simulink model "model2"  (R2023b)
settings: Solver=VariableStepAuto  StartTime=0.0  StopTime=10.0  RelTol=1e-3
undefined symbols (not defined in the file): b1da, d6e66bc8738b, DiscIntNeverNeededParam, magnitude, Newton, Raphson
libraries: simulink x70, slpidlib x25
(part 1 of 4)
settings Model: Creator=OSCAR4  LastModifiedBy=OSCAR4

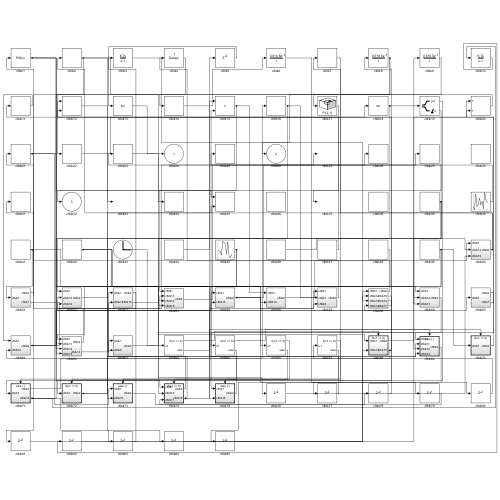
[thumbnail: Simulink's stored preview of the top-level diagram]
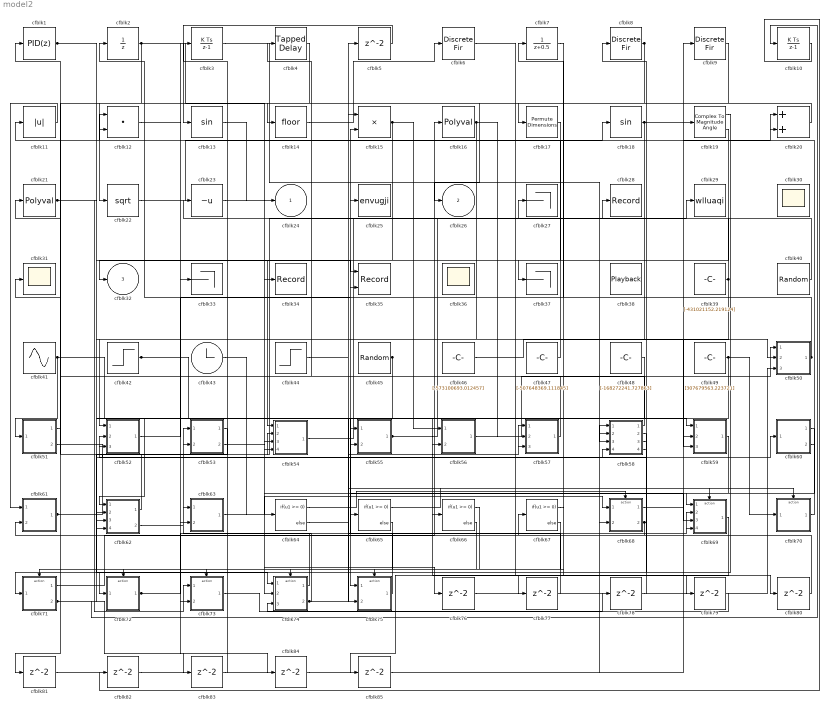
== system model2 ==
  cfblk1 : slpidlib/PID Controller  Controller=PID  Form=Parallel  TimeDomain=Discrete-time  UseExternalTs=off  SampleTime=1  IntegratorMethod=Forward Euler  FilterMethod=Forward Euler  ControllerParametersSource=internal  P=1  I=1  UseKiTs=off  D=0  N=100  UseFilter=on  TunerSelectOption=Transfer Function Based (PID Tuner App)  InitialConditionSource=internal  InitialConditionForIntegrator=0  InitialConditionForFilter=0  DifferentiatorICPrevScaledInput=0  ExternalReset=none  TrackingMode=off  Kt=1  LimitOutput=off  SatLimitsSource=internal  UpperSaturationLimit=inf  LowerSaturationLimit=-inf  LinearizeAsGain=off  AntiWindupMode=none  Kb=1  LimitIntegrator=off  UpperIntegratorSaturationLimit=inf  LowerIntegratorSaturationLimit=-inf  POutMin=[]  POutMax=[]  IOutMin=[]  IOutMax=[]  DOutMin=[]  DOutMax=[]  NOutMin=[]  NOutMax=[]  SumOutMin=[]  SumOutMax=[]  SaturationOutMin=[]  SaturationOutMax=[]  PParamMin=[]  PParamMax=[]  IParamMin=[]  IParamMax=[]  DParamMin=[]  DParamMax=[]  NParamMin=[]  NParamMax=[]  KbParamMin=[]  KbParamMax=[]  KtParamMin=[]  KtParamMax=[]  KbOutMin=[]  KbOutMax=[]  KtOutMin=[]  KtOutMax=[]  IntegratorOutMin=[]  IntegratorOutMax=[]  FilterOutMin=[]  FilterOutMax=[]  SumI1OutMin=[]  SumI1OutMax=[]  SumI2OutMin=[]  SumI2OutMax=[]  SumI3OutMin=[]  SumI3OutMax=[]  SumI4OutMin=[]  SumI4OutMax=[]  SumDOutMin=[]  SumDOutMax=[]  DifferentiatorOutMin=[]  DifferentiatorOutMax=[]  FilterDiffOutCoefMin=[]  FilterDiffOutCoefMax=[]  ReciprocalOutMin=[]  ReciprocalOutMax=[]  SumDenOutMin=[]  SumDenOutMax=[]  SumNumOutMin=[]  SumNumOutMax=[]  DivideOutMin=[]  DivideOutMax=[]  UdiffTsProdOutMin=[]  UdiffTsProdOutMax=[]  NTsProdOutMin=[]  NTsProdOutMax=[]  UintegralTsProdOutMin=[]  UintegralTsProdOutMax=[]  UngainTsProdOutMin=[]  UngainTsProdOutMax=[]  ClampingZeroOutDataTypeStr=Inherit: Inherit via back propagation  ClampingZeroOutMin=[]  ClampingZeroOutMax=[]  FilterDenConstantOutDataTypeStr=Inherit: Inherit via back propagation  FilterDenConstantOutMin=[]  FilterDenConstantOutMax=[]  PCopyOutDataTypeStr=Inherit: Inherit via back propagation  PCopyOutMin=[]  PCopyOutMax=[]  NCopyOutDataTypeStr=Inherit: Inherit via back propagation  NCopyOutMin=[]  NCopyOutMax=[]  IntegratorContinuousStateAttributes=''  IntegratorStateMustResolveToSignalObject=off  IntegratorRTWStateStorageClass=Auto  FilterContinuousStateAttributes=''  FilterStateMustResolveToSignalObject=off  FilterRTWStateStorageClass=Auto  ParallelPVariant=InternalParameters  IdealPVariant=Disabled  IVariant=InternalParameters  DVariant=InternalParameters  IntegratorVariant=Discrete  SatVariant=Disabled  AWVariant=Passthrough  PCopyVariant=Disabled  TRVariant=Disabled  FdbkBlocksVariant=Forward  IdealPFdbkVariant=Disabled  SatFdbkVariant=Disabled  DerivativeFilterVariant=ForwardEulerFilter  NVariant=InternalParameters  NCopyVariant=Disabled  FilterICVariant=InternalICsFilter  IntegratorICVariant=InternalICs  ExternalResetVariant=Disabled  TRSumVariant=Passthrough  SumFdbkVariant=Disabled  SumVariant=Sum_PID  TsampFilterVariant=InternalTs  TsampNgainVariant=Passthrough  TsampIntegralVariant=Disabled_SignalSpec  ExternalSaturationOutDataTypeStr=Inherit: Same as second input
      settings: LibrarySourceBlock=simulink/Discrete/Discrete PID Controller
  cfblk10 : DiscreteIntegrator  ICPrevOutput=DiscIntNeverNeededParam  ICPrevScaledInput=DiscIntNeverNeededParam
  cfblk11 : Abs  SaturateOnIntegerOverflow=off
  cfblk12 : DotProduct  OutDataTypeStr=Inherit: Inherit via internal rule
  cfblk13 : Trigonometry
  cfblk14 : Rounding
  cfblk15 : Product
  cfblk16 : Polyval  Coefs=[ +2.081618890e-019, -1.441693666e-014, +4.719686976e-010, -8.536869453e-006, +1.621573104e-001, -8.087801117e+001 ]
  cfblk17 : PermuteDimensions
  cfblk18 : Trigonometry
  cfblk19 : ComplexToMagnitudeAngle
  cfblk2 : UnitDelay  HasFrameUpgradeWarning=on
  cfblk20 : Sum
  cfblk21 : Polyval  Coefs=[ +2.081618890e-019, -1.441693666e-014, +4.719686976e-010, -8.536869453e-006, +1.621573104e-001, -8.087801117e+001 ]
  cfblk22 : Sqrt
  cfblk23 : UnaryMinus
  cfblk25 : ToWorkspace  VariableName=envugji  SaveFormat=Timeseries  SampleTime=-1
  cfblk27 : Terminator
  cfblk28 : Record  FileSettingsInternal="{\"entries\":[{\"content\":{\"excelSettings\":{\"content\":{},\"type\":\"Streamout.ExcelSettings\"}},\"type\":\"Streamout.FileSettingStorage\",\"uuid\":\"\"}],\"packageUris\":[\"http:\\/\\/schema.mathworks.com\\/mf0\\/streamout_blocks\\/R2020a\"],\"version\":\"1.0\"}"  SignalsInternal="{\"entries\":[{\"content\":{\"signals\":[{\"content\":{\"blockPath\":[],\"dimensions\":[1],\"domain\":\"\",\"lineColor\":\"#ff13a6\",\"plots\":[1],\"port\":1,\"sid\":[\"\"],\"signalID\":1141,\"signalName\":\"cfblk55\"},\"type\":\"RecordBlkView.Signal\",\"uuid\":\"\"}]},\"type\":\"RecordBlkView.InputSignals\",\"uuid\":\"\"}],\"packageUris\":[\"http:\\/\\/schema.mathworks.com\\/mf0\\/streamout_blocks\\/R2020a\"],\"version\":\"1.0\"}"  VisualizationBindings="{\"sparklinesplugin\":{\"info\":[{\"bindingParametersList\":[],\"subplotID\":1}]}}"
  cfblk29 : ToWorkspace  VariableName=wlluaqi  SaveFormat=Timeseries  SampleTime=-1
  cfblk3 : DiscreteIntegrator  ICPrevOutput=DiscIntNeverNeededParam  ICPrevScaledInput=DiscIntNeverNeededParam
  cfblk30 : Scope
      settings: Floating=on
  cfblk31 : Scope
  cfblk33 : Terminator
  cfblk34 : Record  FileSettingsInternal="{\"entries\":[{\"content\":{\"excelSettings\":{\"content\":{},\"type\":\"Streamout.ExcelSettings\"}},\"type\":\"Streamout.FileSettingStorage\",\"uuid\":\"\"}],\"packageUris\":[\"http:\\/\\/schema.mathworks.com\\/mf0\\/streamout_blocks\\/R2020a\"],\"version\":\"1.0\"}"  SignalsInternal="{\"entries\":[{\"content\":{\"signals\":[{\"content\":{\"blockPath\":[],\"dimensions\":[1],\"domain\":\"\",\"lineColor\":\"#22b573\",\"plots\":[1],\"port\":1,\"sid\":[\"\"],\"signalID\":1149,\"signalName\":\"cfblk2\"},\"type\":\"RecordBlkView.Signal\",\"uuid\":\"\"}]},\"type\":\"RecordBlkView.InputSignals\",\"uuid\":\"\"}],\"packageUris\":[\"http:\\/\\/schema.mathworks.com\\/mf0\\/streamout_blocks\\/R2020a\"],\"version\":\"1.0\"}"  VisualizationBindings="{\"sparklinesplugin\":{\"info\":[{\"bindingParametersList\":[],\"subplotID\":1}]}}"
  cfblk35 : Record  FileSettingsInternal="{\"entries\":[{\"content\":{\"excelSettings\":{\"content\":{},\"type\":\"Streamout.ExcelSettings\"}},\"type\":\"Streamout.FileSettingStorage\",\"uuid\":\"\"}],\"packageUris\":[\"http:\\/\\/schema.mathworks.com\\/mf0\\/streamout_blocks\\/R2020a\"],\"version\":\"1.0\"}"  Layout=[1 1]  SignalsInternal="{\"entries\":[{\"content\":{\"signals\":[{\"content\":{\"blockPath\":[],\"dimensions\":[1],\"domain\":\"\",\"lineColor\":\"#a2142f\",\"plots\":[1],\"port\":1,\"sid\":[\"\"],\"signalID\":1153,\"signalName\":\"cfblk1\"},\"type\":\"RecordBlkView.Signal\",\"uuid\":\"\"},{\"content\":{\"blockPath\":[],\"dimensions\":[1],\"domain\":\"\",\"lineColor\":\"#139fff\",\"plots\":[1],\"port\":2,\"sid\":[\"\"],\"signalID\":1157,\"signalName\":\"cfblk52\"},\"type\":\"RecordBlkView.Signal\",\"uuid\":\"\"}]},\"type\":\"RecordBlkView.InputSignals\",\"uuid\":\"\"}],\"packageUris\":[\"http:\\/\\/schema.mathworks.com\\/mf0\\/streamout_blocks\\/R2020a\"],\"version\":\"1.0\"}"  VisualizationBindings="{\"xyplotplugin\":{\"info\":[{\"series\":[{\"bindingParametersList\":[{\"parameter\":\"X-Axis\",\"signalID\":1153,\"signalName\":\"cfblk1\"},{\"parameter\":\"Y-Axis\",\"signalID\":1157,\"signalName\":\"cfblk52\"}],\"seriesID\":35529}],\"subplotID\":1}]}}"  CompatibilityTag=XY
  cfblk36 : Scope
      settings: Floating=on
  cfblk37 : Terminator
  cfblk38 : Playback  NumPorts=0  PartName=63b8ea15-6b82-47df-b1da-d6e66bc8738b
  cfblk39 : Constant  Value=[-431021152.219124]  SampleTime=1
  cfblk4 : simulink/Discrete/Tapped Delay  vinit=0.0  samptime=-1  NumDelays=1  DelayOrder=Oldest  includeCurrent=off
  cfblk40 : UniformRandomNumber  Minimum=[-8305883063.476324]  Maximum=[6336167478.410847]  Seed=[29457914.000000]  SampleTime=0.1
  cfblk41 : Sin  Amplitude=[815797185.839253]  Bias=[956764081.088228]  SampleTime=0
  cfblk42 : Step  Time=[20.000000]  Before=[-203811535.519444]  After=[543324155.345459]  SampleTime=0
  cfblk43 : Clock
  cfblk44 : Step  Time=[32.000000]  Before=[-285476932.662708]  After=[117735768.071794]  SampleTime=0
  cfblk45 : RandomNumber  Mean=[37780.519300]  Variance=[5936.131945]  Seed=[246649944.000000]  SampleTime=0.1
  cfblk46 : Constant  Value=[-573100693.012457]  SampleTime=1
  cfblk47 : Constant  Value=[-507648369.111845]  SampleTime=1
  cfblk48 : Constant  Value=[-168272241.727863]  SampleTime=1
  cfblk49 : Constant  Value=[307679563.223721]  SampleTime=1
  cfblk{5,76..85} (11 alike) : Delay  SampleTime=1
  cfblk50 : Subsystem
  cfblk51 : Subsystem
  cfblk52 : Subsystem
  cfblk53 : Subsystem
  cfblk54 : Subsystem
  cfblk55 : Subsystem
  cfblk56 : Subsystem
  cfblk57 : Subsystem
  cfblk58 : Subsystem
  cfblk59 : Subsystem
  cfblk6 : DiscreteFir  SampleTime=1
  cfblk60 : Subsystem
  cfblk61 : Subsystem
  cfblk62 : Subsystem
  cfblk63 : Subsystem
  cfblk{64..67} (4 alike) : If  IfExpression=u1 >= 0  SampleTime=1
  cfblk68 : Subsystem  TreatAsAtomicUnit=on
  cfblk69 : Subsystem  TreatAsAtomicUnit=on
  cfblk7 : DiscreteTransferFcn  SampleTime=1
  cfblk70 : Subsystem  TreatAsAtomicUnit=on
  cfblk71 : Subsystem  TreatAsAtomicUnit=on
  cfblk72 : Subsystem  TreatAsAtomicUnit=on
  cfblk73 : Subsystem  TreatAsAtomicUnit=on
  cfblk74 : Subsystem  TreatAsAtomicUnit=on
  cfblk75 : Subsystem  TreatAsAtomicUnit=on
  cfblk8 : DiscreteFir  SampleTime=1
  cfblk9 : DiscreteFir  SampleTime=1
  cfblk24 : Outport
  cfblk26 : Outport  Port=2
  cfblk32 : Outport  Port=3
  wires:
  cfblk54/1(cfblk2) -> cfblk29/1
  cfblk14/1 -> cfblk6/1
  cfblk19/1 -> cfblk72/1(cfblk1)
  cfblk41/1 -> cfblk51/1(cfblk1), cfblk56/2(cfblk10)
  cfblk13/1 -> cfblk24/1
  cfblk47/1 -> cfblk11/1
  cfblk21/1 -> cfblk73/1(cfblk1), cfblk74/1(cfblk1)
  cfblk71/1(cfblk2) -> cfblk16/1
  cfblk74/1(cfblk2) -> cfblk53/1(cfblk1)
  cfblk43/1 -> cfblk64/1
  cfblk20/1 -> cfblk17/1
  cfblk62/1(cfblk2) -> cfblk31/1
  cfblk59/1(cfblk2) -> cfblk75/1(cfblk1)
  cfblk56/1(cfblk2) -> cfblk50/1(cfblk1)
  cfblk62/2(cfblk14) -> cfblk53/2(cfblk12)
  cfblk5/1 -> cfblk13/1
  cfblk51/1(cfblk2) -> cfblk1/1
  cfblk4/1 -> cfblk22/1
  cfblk17/1 -> cfblk37/1
  cfblk8/1 -> cfblk26/1, cfblk81/1
  cfblk60/1(cfblk2) -> cfblk69/1(cfblk1)
  cfblk75/1(cfblk2) -> cfblk15/2
  cfblk74/2(cfblk12) -> cfblk63/1(cfblk1), cfblk57/1(cfblk1)
  cfblk3/1 -> cfblk58/3(cfblk13)
  cfblk51/2(cfblk7) -> cfblk60/1(cfblk1)
  cfblk18/1 -> cfblk9/1, cfblk62/3(cfblk12)
  cfblk49/1 -> cfblk65/1, cfblk70/1(cfblk1), cfblk54/3(cfblk14)
  cfblk39/1 -> cfblk52/1(cfblk1), cfblk23/1, cfblk54/4(cfblk15), cfblk59/2(cfblk12)
  cfblk40/1 -> cfblk25/1
  cfblk58/1(cfblk2) -> cfblk21/1
  cfblk72/1(cfblk2) -> cfblk69/2(cfblk11), cfblk69/4(cfblk13)
  cfblk60/2(cfblk7) -> cfblk12/1
  cfblk2/1 -> cfblk33/1, cfblk34/1, cfblk62/2(cfblk11)
  cfblk55/1(cfblk2) -> cfblk28/1, cfblk57/3(cfblk8), cfblk79/1
  cfblk50/1(cfblk2) -> cfblk2/1, cfblk7/1
  cfblk44/1 -> cfblk5/1
  cfblk57/1(cfblk2) -> cfblk4/1
  cfblk61/1(cfblk2) -> cfblk27/1, cfblk54/2(cfblk13), cfblk55/2(cfblk13)
  cfblk42/1 -> cfblk75/2(cfblk16), cfblk66/1, cfblk74/2(cfblk10)
  cfblk46/1 -> cfblk50/2(cfblk14)
  cfblk23/1 -> cfblk69/3(cfblk12)
  cfblk58/2(cfblk15) -> cfblk71/1(cfblk1)
  cfblk58/3(cfblk16) -> cfblk52/2(cfblk15)
  cfblk53/1(cfblk2) -> cfblk52/3(cfblk16)
  cfblk68/1(cfblk2) -> cfblk20/1
  cfblk58/4(cfblk17) -> cfblk12/2
  cfblk15/1 -> cfblk32/1, cfblk56/1(cfblk1)
  cfblk48/1 -> cfblk73/2(cfblk10)
  cfblk1/1 -> cfblk35/1, cfblk59/1(cfblk1), cfblk59/3(cfblk13)
  cfblk11/1 -> cfblk61/1(cfblk1)
  cfblk16/1 -> cfblk63/2(cfblk8), cfblk57/2(cfblk7)
  cfblk19/2 -> cfblk54/1(cfblk1)
  cfblk52/1(cfblk2) -> cfblk35/2
  cfblk45/1 -> cfblk62/1(cfblk1), cfblk62/4(cfblk13)
  cfblk9/1 -> cfblk14/1
  cfblk70/1(cfblk2) -> cfblk20/2
  cfblk68/2(cfblk15) -> cfblk61/2(cfblk12), cfblk8/1
  cfblk63/1(cfblk2) -> cfblk68/1(cfblk1)
  cfblk71/2(cfblk14) -> cfblk10/1, cfblk55/1(cfblk1), cfblk83/1
  cfblk22/1 -> cfblk18/1
  cfblk64/1 -> cfblk68/Action
  cfblk64/2 -> cfblk69/Action
  cfblk65/1 -> cfblk70/Action
  cfblk65/2 -> cfblk71/Action
  cfblk66/1 -> cfblk72/Action
  cfblk66/2 -> cfblk73/Action
  cfblk67/1 -> cfblk74/Action
  cfblk67/2 -> cfblk75/Action
  cfblk53/2(cfblk13) -> cfblk76/1
  cfblk76/1 -> cfblk50/3(cfblk15)
  cfblk7/1 -> cfblk77/1
  cfblk77/1 -> cfblk15/1
  cfblk73/1(cfblk2) -> cfblk78/1
  cfblk78/1 -> cfblk58/4(cfblk14)
  cfblk79/1 -> cfblk74/3(cfblk11)
  cfblk6/1 -> cfblk80/1
  cfblk80/1 -> cfblk67/1
  cfblk81/1 -> cfblk68/2(cfblk14)
  cfblk10/1 -> cfblk82/1
  cfblk82/1 -> cfblk58/2(cfblk12)
  cfblk83/1 -> cfblk3/1
  cfblk12/1 -> cfblk84/1
  cfblk84/1 -> cfblk58/1(cfblk1)
  cfblk69/1(cfblk2) -> cfblk85/1
  cfblk85/1 -> cfblk19/1

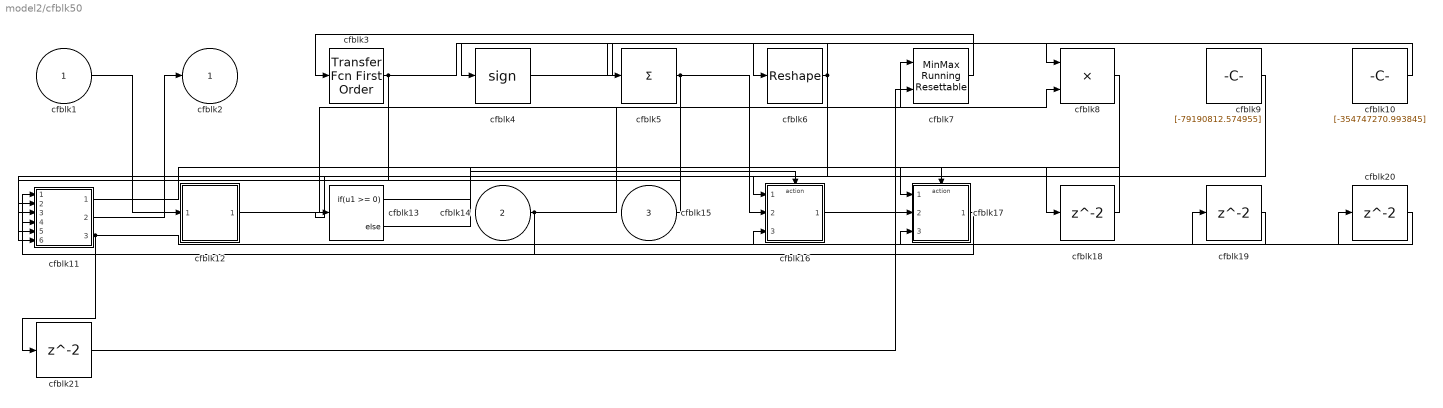
== system model2/cfblk50 ==
  cfblk1 : Inport
  cfblk14 : Inport  Port=2
  cfblk15 : Inport  Port=3
  cfblk10 : Constant  Value=[-354747270.993845]  SampleTime=1
  cfblk11 : Subsystem
  cfblk12 : Subsystem
  cfblk13 : If  IfExpression=u1 >= 0  SampleTime=1
  cfblk16 : Subsystem  TreatAsAtomicUnit=on
  cfblk17 : Subsystem  TreatAsAtomicUnit=on
  cfblk{18..21} (4 alike) : Delay  SampleTime=1
  cfblk3 : simulink/Discrete/Transfer Fcn First Order  PoleZ=0.95  ICPrevOutput=0.0  DoSatur=off
  cfblk4 : Signum
  cfblk5 : Sum  Inputs=+
  cfblk6 : Reshape
  cfblk7 : simulink/Math Operations/MinMax Running Resettable  Function=min  vinit=0.0
  cfblk8 : Product
  cfblk9 : Constant  Value=[-79190812.574955]  SampleTime=1
  cfblk2 : Outport
  wires:
  cfblk1/1 -> cfblk12/1(cfblk1)
  cfblk6/1 -> cfblk4/1, cfblk11/3(cfblk11)
  cfblk12/1(cfblk2) -> cfblk7/1
  cfblk7/1 -> cfblk3/1
  cfblk4/1 -> cfblk8/1
  cfblk10/1 -> cfblk5/1
  cfblk9/1 -> cfblk13/1
  cfblk8/1 -> cfblk16/1(cfblk1)
  cfblk14/1 -> cfblk8/2, cfblk11/4(cfblk12)
  cfblk3/1 -> cfblk6/1, cfblk11/5(cfblk13)
  cfblk17/1(cfblk2) -> cfblk11/1(cfblk1)
  cfblk16/1(cfblk2) -> cfblk17/2(cfblk10)
  cfblk15/1 -> cfblk11/2(cfblk10)
  cfblk5/1 -> cfblk16/2(cfblk10), cfblk11/6(cfblk14)
  cfblk11/2(cfblk15) -> cfblk2/1
  cfblk11/3(cfblk16) -> cfblk19/1, cfblk20/1, cfblk21/1
  cfblk13/1 -> cfblk16/Action
  cfblk13/2 -> cfblk17/Action
  cfblk11/1(cfblk2) -> cfblk18/1
  cfblk18/1 -> cfblk17/1(cfblk1)
  cfblk19/1 -> cfblk16/3(cfblk11)
  cfblk20/1 -> cfblk17/3(cfblk11)
  cfblk21/1 -> cfblk7/2

== system model2/cfblk51 ==
  cfblk1 : Inport
  cfblk3 : Delay  ShowEnablePort=on  SampleTime=1
      settings: InputPortMap=u0,e6
  cfblk4 : Sqrt
  cfblk5 : Sum  Inputs=|++
  cfblk6 : Constant  Value=[536131796.345285]  SampleTime=1
  cfblk8 : Delay  SampleTime=1
  cfblk2 : Outport
  cfblk7 : Outport  Port=2
  wires:
  cfblk6/1 -> cfblk5/1
  cfblk5/1 -> cfblk3/1, cfblk8/1
  cfblk3/1 -> cfblk2/1
  cfblk1/1 -> cfblk3/2
  cfblk4/1 -> cfblk7/1, cfblk5/2
  cfblk8/1 -> cfblk4/1

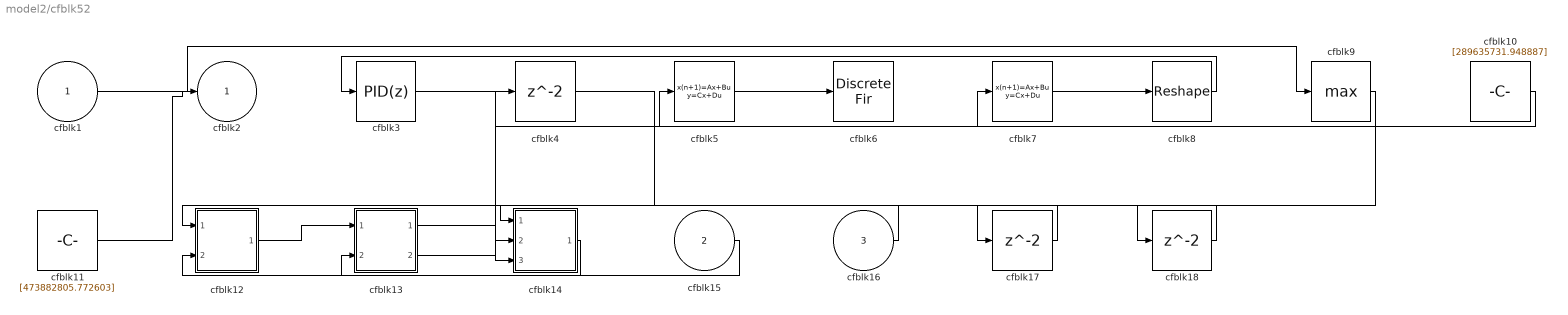
== system model2/cfblk52 ==
  cfblk1 : Inport
  cfblk15 : Inport  Port=2
  cfblk16 : Inport  Port=3
  cfblk10 : Constant  Value=[289635731.948887]  SampleTime=1
  cfblk11 : Constant  Value=[473882805.772603]  SampleTime=1
  cfblk12 : Subsystem
  cfblk13 : Subsystem
  cfblk14 : Subsystem
  cfblk17 : Delay  SampleTime=1
  cfblk18 : Delay  SampleTime=1
  cfblk3 : slpidlib/PID Controller  Controller=PID  Form=Parallel  TimeDomain=Discrete-time  UseExternalTs=off  SampleTime=1  IntegratorMethod=Forward Euler  FilterMethod=Forward Euler  ControllerParametersSource=internal  P=1  I=1  UseKiTs=off  D=0  N=100  UseFilter=on  TunerSelectOption=Transfer Function Based (PID Tuner App)  InitialConditionSource=internal  InitialConditionForIntegrator=0  InitialConditionForFilter=0  DifferentiatorICPrevScaledInput=0  ExternalReset=none  TrackingMode=off  Kt=1  LimitOutput=off  SatLimitsSource=internal  UpperSaturationLimit=inf  LowerSaturationLimit=-inf  LinearizeAsGain=off  AntiWindupMode=none  Kb=1  LimitIntegrator=off  UpperIntegratorSaturationLimit=inf  LowerIntegratorSaturationLimit=-inf  POutMin=[]  POutMax=[]  IOutMin=[]  IOutMax=[]  DOutMin=[]  DOutMax=[]  NOutMin=[]  NOutMax=[]  SumOutMin=[]  SumOutMax=[]  SaturationOutMin=[]  SaturationOutMax=[]  PParamMin=[]  PParamMax=[]  IParamMin=[]  IParamMax=[]  DParamMin=[]  DParamMax=[]  NParamMin=[]  NParamMax=[]  KbParamMin=[]  KbParamMax=[]  KtParamMin=[]  KtParamMax=[]  KbOutMin=[]  KbOutMax=[]  KtOutMin=[]  KtOutMax=[]  IntegratorOutMin=[]  IntegratorOutMax=[]  FilterOutMin=[]  FilterOutMax=[]  SumI1OutMin=[]  SumI1OutMax=[]  SumI2OutMin=[]  SumI2OutMax=[]  SumI3OutMin=[]  SumI3OutMax=[]  SumI4OutMin=[]  SumI4OutMax=[]  SumDOutMin=[]  SumDOutMax=[]  DifferentiatorOutMin=[]  DifferentiatorOutMax=[]  FilterDiffOutCoefMin=[]  FilterDiffOutCoefMax=[]  ReciprocalOutMin=[]  ReciprocalOutMax=[]  SumDenOutMin=[]  SumDenOutMax=[]  SumNumOutMin=[]  SumNumOutMax=[]  DivideOutMin=[]  DivideOutMax=[]  UdiffTsProdOutMin=[]  UdiffTsProdOutMax=[]  NTsProdOutMin=[]  NTsProdOutMax=[]  UintegralTsProdOutMin=[]  UintegralTsProdOutMax=[]  UngainTsProdOutMin=[]  UngainTsProdOutMax=[]  ClampingZeroOutDataTypeStr=Inherit: Inherit via back propagation  ClampingZeroOutMin=[]  ClampingZeroOutMax=[]  FilterDenConstantOutDataTypeStr=Inherit: Inherit via back propagation  FilterDenConstantOutMin=[]  FilterDenConstantOutMax=[]  PCopyOutDataTypeStr=Inherit: Inherit via back propagation  PCopyOutMin=[]  PCopyOutMax=[]  NCopyOutDataTypeStr=Inherit: Inherit via back propagation  NCopyOutMin=[]  NCopyOutMax=[]  IntegratorContinuousStateAttributes=''  IntegratorStateMustResolveToSignalObject=off  IntegratorRTWStateStorageClass=Auto  FilterContinuousStateAttributes=''  FilterStateMustResolveToSignalObject=off  FilterRTWStateStorageClass=Auto  ParallelPVariant=InternalParameters  IdealPVariant=Disabled  IVariant=InternalParameters  DVariant=InternalParameters  IntegratorVariant=Discrete  SatVariant=Disabled  AWVariant=Passthrough  PCopyVariant=Disabled  TRVariant=Disabled  FdbkBlocksVariant=Forward  IdealPFdbkVariant=Disabled  SatFdbkVariant=Disabled  DerivativeFilterVariant=ForwardEulerFilter  NVariant=InternalParameters  NCopyVariant=Disabled  FilterICVariant=InternalICsFilter  IntegratorICVariant=InternalICs  ExternalResetVariant=Disabled  TRSumVariant=Passthrough  SumFdbkVariant=Disabled  SumVariant=Sum_PID  TsampFilterVariant=InternalTs  TsampNgainVariant=Passthrough  TsampIntegralVariant=Disabled_SignalSpec  ExternalSaturationOutDataTypeStr=Inherit: Same as second input
      settings: LibrarySourceBlock=simulink/Discrete/Discrete PID Controller
  cfblk4 : Delay  SampleTime=1
  cfblk5 : DiscreteStateSpace
  cfblk6 : DiscreteFir  SampleTime=1
  cfblk7 : DiscreteStateSpace
  cfblk8 : Reshape
  cfblk9 : MinMax  Function=max
  cfblk2 : Outport
  wires:
  cfblk16/1 -> cfblk12/1(cfblk1)
  cfblk8/1 -> cfblk3/1
  cfblk5/1 -> cfblk6/1
  cfblk7/1 -> cfblk8/1
  cfblk12/1(cfblk2) -> cfblk13/1(cfblk1)
  cfblk1/1 -> cfblk9/1
  cfblk10/1 -> cfblk5/1
  cfblk9/1 -> cfblk14/3(cfblk9)
  cfblk11/1 -> cfblk2/1
  cfblk14/1(cfblk2) -> cfblk12/2(cfblk7)
  cfblk15/1 -> cfblk13/2(cfblk13)
  cfblk13/1(cfblk2) -> cfblk4/1
  cfblk13/2(cfblk14) -> cfblk7/1
  cfblk4/1 -> cfblk17/1
  cfblk17/1 -> cfblk14/2(cfblk8)
  cfblk3/1 -> cfblk18/1
  cfblk18/1 -> cfblk14/1(cfblk1)

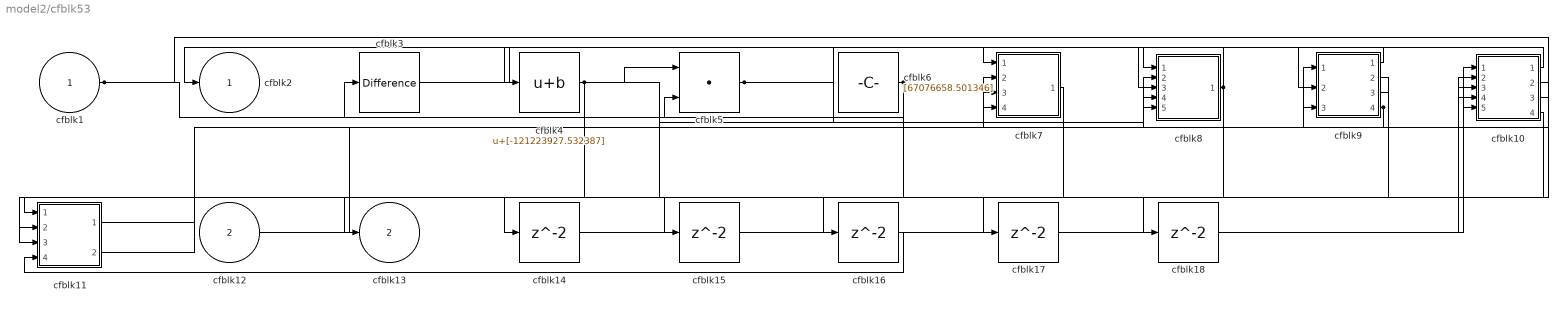
== system model2/cfblk53 ==
  cfblk1 : Inport
  cfblk12 : Inport  Port=2
  cfblk10 : Subsystem
  cfblk11 : Subsystem
  cfblk{14..18} (5 alike) : Delay  SampleTime=1
  cfblk3 : simulink/Discrete/Difference  ICPrevInput=0.0  OutMin=[]  OutMax=[]  OutDataTypeStr=Inherit: Inherit via back propagation  OutDataType=fixdt(1, 16)  OutScaling=2^-10  DoSatur=off
  cfblk4 : Bias  Bias=[-121223927.532387]  SaturateOnIntegerOverflow=off
  cfblk5 : DotProduct  OutDataTypeStr=Inherit: Inherit via internal rule
  cfblk6 : Constant  Value=[67076658.501346]  SampleTime=1
  cfblk7 : Subsystem
  cfblk8 : Subsystem
  cfblk9 : Subsystem
  cfblk2 : Outport
  cfblk13 : Outport  Port=2
  wires:
  cfblk4/1 -> cfblk5/1, cfblk13/1, cfblk8/4(cfblk7), cfblk17/1
  cfblk12/1 -> cfblk9/1(cfblk1)
  cfblk8/1(cfblk2) -> cfblk2/1, cfblk16/1
  cfblk10/1(cfblk2) -> cfblk7/1(cfblk1)
  cfblk6/1 -> cfblk3/1, cfblk11/3(cfblk13)
  cfblk3/1 -> cfblk9/2(cfblk13)
  cfblk1/1 -> cfblk10/1(cfblk1), cfblk5/2
  cfblk10/2(cfblk15) -> cfblk11/1(cfblk1)
  cfblk10/3(cfblk16) -> cfblk7/2(cfblk13)
  cfblk5/1 -> cfblk8/1(cfblk1), cfblk8/3(cfblk6), cfblk8/5(cfblk8)
  cfblk11/2(cfblk15) -> cfblk9/3(cfblk14)
  cfblk10/4(cfblk17) -> cfblk11/2(cfblk12)
  cfblk9/1(cfblk2) -> cfblk4/1
  cfblk9/3(cfblk16) -> cfblk7/3(cfblk14)
  cfblk9/4(cfblk17) -> cfblk8/2(cfblk5), cfblk7/4(cfblk15)
  cfblk7/1(cfblk2) -> cfblk14/1
  cfblk14/1 -> cfblk10/2(cfblk11)
  cfblk11/1(cfblk2) -> cfblk15/1
  cfblk15/1 -> cfblk10/3(cfblk12)
  cfblk16/1 -> cfblk11/4(cfblk14)
  cfblk17/1 -> cfblk10/5(cfblk14)
  cfblk9/2(cfblk15) -> cfblk18/1
  cfblk18/1 -> cfblk10/4(cfblk13)

== system model2/cfblk54 ==
  cfblk1 : Inport
  cfblk13 : Inport  Port=2
  cfblk14 : Inport  Port=3
  cfblk15 : Inport  Port=4
  cfblk10 : Subsystem
  cfblk11 : Subsystem
  cfblk12 : Subsystem
  cfblk16 : Delay  SampleTime=1
  cfblk17 : Delay  SampleTime=1
  cfblk3 : DiscreteStateSpace
  cfblk4 : simulink/Discrete/Transfer Fcn Lead or Lag  PoleZ=0.95  ZeroZ=0.75  ICPrevOutput=0.0  ICPrevInput=0.0  DoSatur=off
  cfblk5 : Trigonometry
  cfblk6 : ComplexToRealImag
  cfblk7 : Constant  Value=[-514549736.041754]  SampleTime=1
  cfblk8 : Subsystem
  cfblk9 : Subsystem
  cfblk2 : Outport
  wires:
  cfblk13/1 -> cfblk3/1
  cfblk10/1(cfblk2) -> cfblk5/1
  cfblk5/1 -> cfblk6/1
  cfblk1/1 -> cfblk12/1(cfblk1)
  cfblk4/1 -> cfblk8/1(cfblk1)
  cfblk12/1(cfblk2) -> cfblk10/2(cfblk8)
  cfblk11/1(cfblk2) -> cfblk9/1(cfblk1)
  cfblk3/1 -> cfblk9/2(cfblk7)
  cfblk6/1 -> cfblk11/1(cfblk1)
  cfblk6/2 -> cfblk2/1
  cfblk11/2(cfblk16) -> cfblk9/3(cfblk8)
  cfblk14/1 -> cfblk12/2(cfblk7)
  cfblk15/1 -> cfblk9/4(cfblk9)
  cfblk7/1 -> cfblk11/2(cfblk14)
  cfblk12/2(cfblk8) -> cfblk11/3(cfblk15)
  cfblk9/1(cfblk2) -> cfblk16/1
  cfblk16/1 -> cfblk10/1(cfblk1)
  cfblk8/1(cfblk2) -> cfblk17/1
  cfblk17/1 -> cfblk4/1

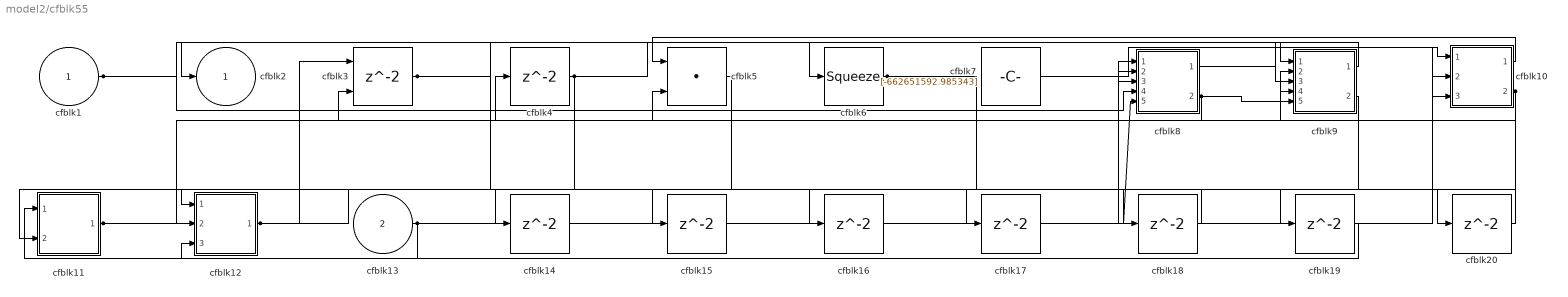
== system model2/cfblk55 ==
  cfblk1 : Inport
  cfblk13 : Inport  Port=2
  cfblk10 : Subsystem
  cfblk11 : Subsystem
  cfblk12 : Subsystem
  cfblk{4,14..20} (8 alike) : Delay  SampleTime=1
  cfblk3 : Delay  ShowEnablePort=on  SampleTime=1
      settings: InputPortMap=u0,e6
  cfblk5 : DotProduct  OutDataTypeStr=Inherit: Inherit via internal rule
  cfblk6 : Squeeze
  cfblk7 : Constant  Value=[-662651592.985343]  SampleTime=1
  cfblk8 : Subsystem
  cfblk9 : Subsystem
  cfblk2 : Outport
  wires:
  cfblk7/1 -> cfblk10/1(cfblk1)
  cfblk6/1 -> cfblk18/1, cfblk19/1
  cfblk10/1(cfblk2) -> cfblk5/1
  cfblk11/1(cfblk2) -> cfblk9/4(cfblk10), cfblk20/1
  cfblk4/1 -> cfblk9/1(cfblk1), cfblk11/2(cfblk8)
  cfblk9/1(cfblk2) -> cfblk2/1
  cfblk8/1(cfblk2) -> cfblk10/3(cfblk12)
  cfblk10/2(cfblk13) -> cfblk9/2(cfblk8), cfblk12/2(cfblk12), cfblk3/2
  cfblk8/2(cfblk16) -> cfblk5/2, cfblk9/5(cfblk11)
  cfblk12/1(cfblk2) -> cfblk3/1, cfblk16/1
  cfblk3/1 -> cfblk6/1, cfblk17/1
  cfblk13/1 -> cfblk11/1(cfblk1), cfblk8/5(cfblk15)
  cfblk1/1 -> cfblk8/4(cfblk14), cfblk9/3(cfblk9)
  cfblk5/1 -> cfblk14/1
  cfblk14/1 -> cfblk10/2(cfblk11)
  cfblk9/2(cfblk12) -> cfblk15/1
  cfblk15/1 -> cfblk8/3(cfblk13)
  cfblk16/1 -> cfblk8/1(cfblk1)
  cfblk17/1 -> cfblk8/2(cfblk12)
  cfblk18/1 -> cfblk12/1(cfblk1)
  cfblk19/1 -> cfblk12/3(cfblk13)
  cfblk20/1 -> cfblk4/1

== system model2/cfblk56 ==
  cfblk1 : Inport
  cfblk10 : Inport  Port=2
  cfblk{11..14} (4 alike) : Delay  SampleTime=1
  cfblk3 : DiscreteFir  SampleTime=1
  cfblk4 : Rounding
  cfblk5 : Sin  TimeSource=Use external signal  SampleTime=0
  cfblk6 : Assignment  DiagnosticForDimensions=Warning  IndexOptions=Index vector (dialog)  Indices=1  OutputSizes=1
  cfblk7 : Polyval  Coefs=[ +2.081618890e-019, -1.441693666e-014, +4.719686976e-010, -8.536869453e-006, +1.621573104e-001, -8.087801117e+001 ]
  cfblk8 : Subsystem
  cfblk9 : Subsystem
  cfblk2 : Outport
  wires:
  cfblk4/1 -> cfblk6/1, cfblk12/1, cfblk13/1
  cfblk10/1 -> cfblk2/1
  cfblk8/1(cfblk2) -> cfblk5/1
  cfblk7/1 -> cfblk3/1, cfblk8/3(cfblk8)
  cfblk1/1 -> cfblk7/1
  cfblk5/1 -> cfblk4/1
  cfblk9/1(cfblk2) -> cfblk6/2
  cfblk3/1 -> cfblk9/2(cfblk6), cfblk8/5(cfblk10)
  cfblk9/2(cfblk8) -> cfblk8/1(cfblk1), cfblk8/6(cfblk11)
  cfblk6/1 -> cfblk11/1
  cfblk11/1 -> cfblk9/1(cfblk1)
  cfblk12/1 -> cfblk8/2(cfblk7)
  cfblk13/1 -> cfblk8/4(cfblk9)
  cfblk8/2(cfblk12) -> cfblk14/1
  cfblk14/1 -> cfblk9/3(cfblk7)

== system model2/cfblk57 ==
  cfblk1 : Inport
  cfblk7 : Inport  Port=2
  cfblk8 : Inport  Port=3
  cfblk10 : Subsystem  TreatAsAtomicUnit=on
  cfblk{11..15} (5 alike) : Delay  SampleTime=1
  cfblk3 : Product  Inputs=*
  cfblk4 : Subsystem
  cfblk5 : Subsystem
  cfblk6 : If  IfExpression=u1 >= 0  SampleTime=1
  cfblk9 : Subsystem  TreatAsAtomicUnit=on
  cfblk2 : Outport
  wires:
  cfblk8/1 -> cfblk2/1, cfblk5/3(cfblk12)
  cfblk1/1 -> cfblk5/1(cfblk1)
  cfblk9/1(cfblk2) -> cfblk10/1(cfblk1)
  cfblk7/1 -> cfblk9/2(cfblk9)
  cfblk10/1(cfblk2) -> cfblk3/1, cfblk11/1, cfblk15/1
  cfblk3/1 -> cfblk4/1(cfblk1), cfblk4/3(cfblk7), cfblk4/6(cfblk10)
  cfblk5/1(cfblk2) -> cfblk9/4(cfblk11)
  cfblk5/2(cfblk14) -> cfblk10/3(cfblk11)
  cfblk5/3(cfblk15) -> cfblk6/1, cfblk4/2(cfblk6), cfblk4/4(cfblk8), cfblk4/5(cfblk9)
  cfblk6/1 -> cfblk9/Action
  cfblk6/2 -> cfblk10/Action
  cfblk11/1 -> cfblk9/3(cfblk10)
  cfblk4/1(cfblk2) -> cfblk12/1
  cfblk12/1 -> cfblk9/1(cfblk1)
  cfblk4/2(cfblk11) -> cfblk13/1
  cfblk13/1 -> cfblk10/2(cfblk10)
  cfblk4/3(cfblk12) -> cfblk14/1
  cfblk14/1 -> cfblk5/2(cfblk11)
  cfblk15/1 -> cfblk5/4(cfblk13)

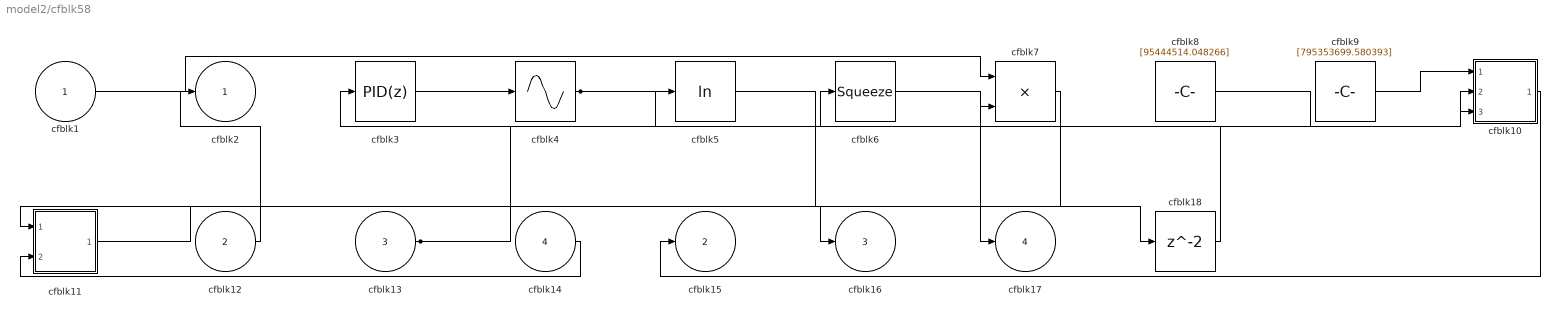
== system model2/cfblk58 ==
  cfblk1 : Inport
  cfblk12 : Inport  Port=2
  cfblk13 : Inport  Port=3
  cfblk14 : Inport  Port=4
  cfblk10 : Subsystem
  cfblk11 : Subsystem
  cfblk18 : Delay  SampleTime=1
  cfblk3 : slpidlib/PID Controller  Controller=PID  Form=Parallel  TimeDomain=Discrete-time  UseExternalTs=off  SampleTime=1  IntegratorMethod=Forward Euler  FilterMethod=Forward Euler  ControllerParametersSource=internal  P=1  I=1  UseKiTs=off  D=0  N=100  UseFilter=on  TunerSelectOption=Transfer Function Based (PID Tuner App)  InitialConditionSource=internal  InitialConditionForIntegrator=0  InitialConditionForFilter=0  DifferentiatorICPrevScaledInput=0  ExternalReset=none  TrackingMode=off  Kt=1  LimitOutput=off  SatLimitsSource=internal  UpperSaturationLimit=inf  LowerSaturationLimit=-inf  LinearizeAsGain=off  AntiWindupMode=none  Kb=1  LimitIntegrator=off  UpperIntegratorSaturationLimit=inf  LowerIntegratorSaturationLimit=-inf  POutMin=[]  POutMax=[]  IOutMin=[]  IOutMax=[]  DOutMin=[]  DOutMax=[]  NOutMin=[]  NOutMax=[]  SumOutMin=[]  SumOutMax=[]  SaturationOutMin=[]  SaturationOutMax=[]  PParamMin=[]  PParamMax=[]  IParamMin=[]  IParamMax=[]  DParamMin=[]  DParamMax=[]  NParamMin=[]  NParamMax=[]  KbParamMin=[]  KbParamMax=[]  KtParamMin=[]  KtParamMax=[]  KbOutMin=[]  KbOutMax=[]  KtOutMin=[]  KtOutMax=[]  IntegratorOutMin=[]  IntegratorOutMax=[]  FilterOutMin=[]  FilterOutMax=[]  SumI1OutMin=[]  SumI1OutMax=[]  SumI2OutMin=[]  SumI2OutMax=[]  SumI3OutMin=[]  SumI3OutMax=[]  SumI4OutMin=[]  SumI4OutMax=[]  SumDOutMin=[]  SumDOutMax=[]  DifferentiatorOutMin=[]  DifferentiatorOutMax=[]  FilterDiffOutCoefMin=[]  FilterDiffOutCoefMax=[]  ReciprocalOutMin=[]  ReciprocalOutMax=[]  SumDenOutMin=[]  SumDenOutMax=[]  SumNumOutMin=[]  SumNumOutMax=[]  DivideOutMin=[]  DivideOutMax=[]  UdiffTsProdOutMin=[]  UdiffTsProdOutMax=[]  NTsProdOutMin=[]  NTsProdOutMax=[]  UintegralTsProdOutMin=[]  UintegralTsProdOutMax=[]  UngainTsProdOutMin=[]  UngainTsProdOutMax=[]  ClampingZeroOutDataTypeStr=Inherit: Inherit via back propagation  ClampingZeroOutMin=[]  ClampingZeroOutMax=[]  FilterDenConstantOutDataTypeStr=Inherit: Inherit via back propagation  FilterDenConstantOutMin=[]  FilterDenConstantOutMax=[]  PCopyOutDataTypeStr=Inherit: Inherit via back propagation  PCopyOutMin=[]  PCopyOutMax=[]  NCopyOutDataTypeStr=Inherit: Inherit via back propagation  NCopyOutMin=[]  NCopyOutMax=[]  IntegratorContinuousStateAttributes=''  IntegratorStateMustResolveToSignalObject=off  IntegratorRTWStateStorageClass=Auto  FilterContinuousStateAttributes=''  FilterStateMustResolveToSignalObject=off  FilterRTWStateStorageClass=Auto  ParallelPVariant=InternalParameters  IdealPVariant=Disabled  IVariant=InternalParameters  DVariant=InternalParameters  IntegratorVariant=Discrete  SatVariant=Disabled  AWVariant=Passthrough  PCopyVariant=Disabled  TRVariant=Disabled  FdbkBlocksVariant=Forward  IdealPFdbkVariant=Disabled  SatFdbkVariant=Disabled  DerivativeFilterVariant=ForwardEulerFilter  NVariant=InternalParameters  NCopyVariant=Disabled  FilterICVariant=InternalICsFilter  IntegratorICVariant=InternalICs  ExternalResetVariant=Disabled  TRSumVariant=Passthrough  SumFdbkVariant=Disabled  SumVariant=Sum_PID  TsampFilterVariant=InternalTs  TsampNgainVariant=Passthrough  TsampIntegralVariant=Disabled_SignalSpec  ExternalSaturationOutDataTypeStr=Inherit: Same as second input
      settings: LibrarySourceBlock=simulink/Discrete/Discrete PID Controller
  cfblk4 : Sin  TimeSource=Use external signal  SampleTime=0
  cfblk5 : Math  Operator=log
  cfblk6 : Squeeze
  cfblk7 : Product
  cfblk8 : Constant  Value=[95444514.048266]  SampleTime=1
  cfblk9 : Constant  Value=[795353699.580393]  SampleTime=1
  cfblk2 : Outport
  cfblk15 : Outport  Port=2
  cfblk16 : Outport  Port=3
  cfblk17 : Outport  Port=4
  wires:
  cfblk7/1 -> cfblk11/1(cfblk1)
  cfblk10/1(cfblk2) -> cfblk15/1
  cfblk14/1 -> cfblk11/2(cfblk8)
  cfblk6/1 -> cfblk17/1
  cfblk3/1 -> cfblk4/1
  cfblk9/1 -> cfblk10/1(cfblk1)
  cfblk1/1 -> cfblk7/1
  cfblk12/1 -> cfblk2/1
  cfblk4/1 -> cfblk5/1, cfblk7/2
  cfblk11/1(cfblk2) -> cfblk16/1
  cfblk8/1 -> cfblk10/2(cfblk14)
  cfblk13/1 -> cfblk10/3(cfblk15), cfblk6/1
  cfblk5/1 -> cfblk18/1
  cfblk18/1 -> cfblk3/1

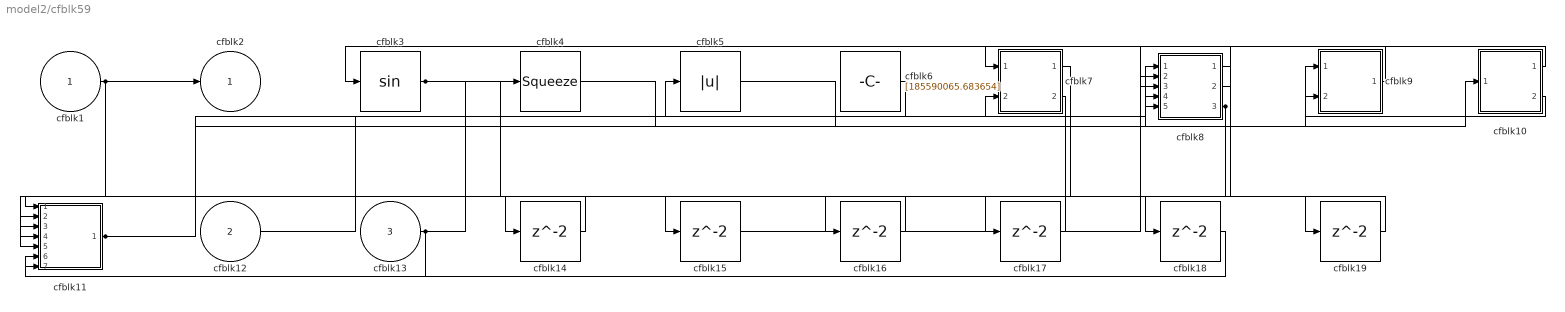
== system model2/cfblk59 ==
  cfblk1 : Inport
  cfblk12 : Inport  Port=2
  cfblk13 : Inport  Port=3
  cfblk10 : Subsystem
  cfblk11 : Subsystem
  cfblk{14..19} (6 alike) : Delay  SampleTime=1
  cfblk3 : Trigonometry
  cfblk4 : Squeeze
  cfblk5 : Abs  SaturateOnIntegerOverflow=off
  cfblk6 : Constant  Value=[185590065.683654]  SampleTime=1
  cfblk7 : Subsystem
  cfblk8 : Subsystem
  cfblk9 : Subsystem
  cfblk2 : Outport
  wires:
  cfblk13/1 -> cfblk4/1, cfblk11/6(cfblk13)
  cfblk1/1 -> cfblk2/1, cfblk11/5(cfblk12)
  cfblk10/1(cfblk2) -> cfblk3/1
  cfblk6/1 -> cfblk5/1
  cfblk10/2(cfblk8) -> cfblk9/1(cfblk1)
  cfblk4/1 -> cfblk8/1(cfblk1)
  cfblk5/1 -> cfblk9/2(cfblk11)
  cfblk9/1(cfblk2) -> cfblk8/3(cfblk12)
  cfblk8/2(cfblk15) -> cfblk7/1(cfblk1)
  cfblk11/1(cfblk2) -> cfblk8/4(cfblk13), cfblk10/1(cfblk1)
  cfblk8/3(cfblk16) -> cfblk17/1, cfblk18/1
  cfblk12/1 -> cfblk8/5(cfblk14)
  cfblk3/1 -> cfblk7/2(cfblk12), cfblk19/1
  cfblk8/1(cfblk2) -> cfblk14/1
  cfblk14/1 -> cfblk11/1(cfblk1)
  cfblk7/1(cfblk2) -> cfblk15/1
  cfblk15/1 -> cfblk8/2(cfblk11)
  cfblk7/2(cfblk13) -> cfblk16/1
  cfblk16/1 -> cfblk11/2(cfblk9)
  cfblk17/1 -> cfblk11/3(cfblk10)
  cfblk18/1 -> cfblk11/7(cfblk14)
  cfblk19/1 -> cfblk11/4(cfblk11)

== system model2/cfblk60 ==
  cfblk1 : Inport
  cfblk3 : UnitDelay  HasFrameUpgradeWarning=on
  cfblk4 : Abs  SaturateOnIntegerOverflow=off
  cfblk5 : simulink/Math Operations/Slider Gain  gain=1  low=0  high=2
  cfblk6 : Subsystem
  cfblk8 : Delay  SampleTime=1
  cfblk2 : Outport
  cfblk7 : Outport  Port=2
  wires:
  cfblk5/1 -> cfblk7/1
  cfblk1/1 -> cfblk5/1, cfblk6/2(cfblk12)
  cfblk6/1(cfblk2) -> cfblk3/1
  cfblk6/2(cfblk13) -> cfblk2/1
  cfblk3/1 -> cfblk4/1
  cfblk4/1 -> cfblk8/1
  cfblk8/1 -> cfblk6/1(cfblk1)

== system model2/cfblk61 ==
  cfblk1 : Inport
  cfblk12 : Inport  Port=2
  cfblk10 : Constant  Value=[389037315.752305]  SampleTime=1
  cfblk11 : Subsystem
  cfblk3 : simulink/Discrete/Difference  ICPrevInput=0.0  OutMin=[]  OutMax=[]  OutDataTypeStr=Inherit: Inherit via back propagation  OutDataType=fixdt(1, 16)  OutScaling=2^-10  DoSatur=off
  cfblk4 : DiscreteIntegrator  ICPrevOutput=DiscIntNeverNeededParam  ICPrevScaledInput=DiscIntNeverNeededParam
  cfblk5 : Abs  SaturateOnIntegerOverflow=off
  cfblk6 : Polyval  Coefs=[ +2.081618890e-019, -1.441693666e-014, +4.719686976e-010, -8.536869453e-006, +1.621573104e-001, -8.087801117e+001 ]
  cfblk7 : Sum  Inputs=+-
  cfblk8 : Abs  SaturateOnIntegerOverflow=off
  cfblk9 : Product  Inputs=**
  cfblk2 : Outport
  wires:
  cfblk1/1 -> cfblk8/1
  cfblk6/1 -> cfblk5/1
  cfblk10/1 -> cfblk6/1
  cfblk12/1 -> cfblk7/1, cfblk7/2
  cfblk4/1 -> cfblk9/1
  cfblk3/1 -> cfblk4/1
  cfblk5/1 -> cfblk3/1
  cfblk8/1 -> cfblk11/1(cfblk1), cfblk11/3(cfblk8)
  cfblk11/1(cfblk2) -> cfblk9/2
  cfblk7/1 -> cfblk11/2(cfblk7), cfblk11/4(cfblk9)
  cfblk9/1 -> cfblk2/1

== system model2/cfblk62 ==
  cfblk1 : Inport
  cfblk11 : Inport  Port=2
  cfblk12 : Inport  Port=3
  cfblk13 : Inport  Port=4
  cfblk10 : Subsystem
  cfblk15 : Delay  SampleTime=1
  cfblk16 : Delay  SampleTime=1
  cfblk3 : Rounding
  cfblk4 : Rounding
  cfblk5 : Bias  Bias=[551164173.250226]  SaturateOnIntegerOverflow=off
  cfblk6 : Rounding
  cfblk7 : Polyval  Coefs=[ +2.081618890e-019, -1.441693666e-014, +4.719686976e-010, -8.536869453e-006, +1.621573104e-001, -8.087801117e+001 ]
  cfblk8 : PermuteDimensions
  cfblk9 : Gain  Gain=[323688973.349032]
  cfblk2 : Outport
  cfblk14 : Outport  Port=2
  wires:
  cfblk10/1(cfblk2) -> cfblk14/1
  cfblk9/1 -> cfblk4/1
  cfblk10/2(cfblk12) -> cfblk2/1
  cfblk6/1 -> cfblk8/1
  cfblk5/1 -> cfblk7/1
  cfblk10/3(cfblk13) -> cfblk9/1
  cfblk12/1 -> cfblk3/1
  cfblk1/1 -> cfblk10/1(cfblk1)
  cfblk3/1 -> cfblk10/2(cfblk11)
  cfblk7/1 -> cfblk15/1
  cfblk15/1 -> cfblk5/1
  cfblk8/1 -> cfblk16/1
  cfblk16/1 -> cfblk6/1

== system model2/cfblk63 ==
  cfblk1 : Inport
  cfblk8 : Inport  Port=2
  cfblk10 : Delay  SampleTime=1
  cfblk11 : Delay  SampleTime=1
  cfblk3 : slpidlib/PID Controller (2DOF)  Controller=PID  Form=Parallel  TimeDomain=Discrete-time  UseExternalTs=off  SampleTime=1  IntegratorMethod=Forward Euler  FilterMethod=Forward Euler  ControllerParametersSource=internal  P=1  I=1  UseKiTs=off  D=0  N=100  UseFilter=on  b=1  c=1  TunerSelectOption=Transfer Function Based (PID Tuner App)  InitialConditionSource=internal  InitialConditionForIntegrator=0  InitialConditionForFilter=0  DifferentiatorICPrevScaledInput=0  ExternalReset=none  TrackingMode=off  Kt=1  LimitOutput=off  SatLimitsSource=internal  UpperSaturationLimit=inf  LowerSaturationLimit=-inf  LinearizeAsGain=off  AntiWindupMode=none  Kb=1  LimitIntegrator=off  UpperIntegratorSaturationLimit=inf  LowerIntegratorSaturationLimit=-inf  POutMin=[]  POutMax=[]  IOutMin=[]  IOutMax=[]  DOutMin=[]  DOutMax=[]  NOutMin=[]  NOutMax=[]  bOutMin=[]  bOutMax=[]  cOutMin=[]  cOutMax=[]  SumOutMin=[]  SumOutMax=[]  SaturationOutMin=[]  SaturationOutMax=[]  PParamMin=[]  PParamMax=[]  IParamMin=[]  IParamMax=[]  DParamMin=[]  DParamMax=[]  NParamMin=[]  NParamMax=[]  bParamMin=[]  bParamMax=[]  cParamMin=[]  cParamMax=[]  KbParamMin=[]  KbParamMax=[]  KtParamMin=[]  KtParamMax=[]  KbOutMin=[]  KbOutMax=[]  KtOutMin=[]  KtOutMax=[]  IntegratorOutMin=[]  IntegratorOutMax=[]  FilterOutMin=[]  FilterOutMax=[]  SumI1OutMin=[]  SumI1OutMax=[]  SumI2OutMin=[]  SumI2OutMax=[]  SumI3OutMin=[]  SumI3OutMax=[]  SumI4OutMin=[]  SumI4OutMax=[]  SumDOutMin=[]  SumDOutMax=[]  Sum1OutMin=[]  Sum1OutMax=[]  Sum2OutMin=[]  Sum2OutMax=[]  Sum3OutMin=[]  Sum3OutMax=[]  DifferentiatorOutMin=[]  DifferentiatorOutMax=[]  FilterDiffOutCoefMin=[]  FilterDiffOutCoefMax=[]  ReciprocalOutMin=[]  ReciprocalOutMax=[]  SumDenOutMin=[]  SumDenOutMax=[]  SumNumOutMin=[]  SumNumOutMax=[]  DivideOutMin=[]  DivideOutMax=[]  UdiffTsProdOutMin=[]  UdiffTsProdOutMax=[]  NTsProdOutMin=[]  NTsProdOutMax=[]  UintegralTsProdOutMin=[]  UintegralTsProdOutMax=[]  UngainTsProdOutMin=[]  UngainTsProdOutMax=[]  ClampingZeroOutDataTypeStr=Inherit: Inherit via back propagation  ClampingZeroOutMin=[]  ClampingZeroOutMax=[]  FilterDenConstantOutDataTypeStr=Inherit: Inherit via back propagation  FilterDenConstantOutMin=[]  FilterDenConstantOutMax=[]  PCopyOutDataTypeStr=Inherit: Inherit via back propagation  PCopyOutMin=[]  PCopyOutMax=[]  NCopyOutDataTypeStr=Inherit: Inherit via back propagation  NCopyOutMin=[]  NCopyOutMax=[]  IntegratorContinuousStateAttributes=''  IntegratorStateMustResolveToSignalObject=off  IntegratorRTWStateStorageClass=Auto  FilterContinuousStateAttributes=''  FilterStateMustResolveToSignalObject=off  FilterRTWStateStorageClass=Auto  ParallelPVariant=InternalParameters  IdealPVariant=Disabled  IVariant=InternalParameters  DVariant=InternalParameters  bVariant=InternalParameters  cVariant=InternalParameters  IntegratorVariant=Discrete  SatVariant=Disabled  AWVariant=Passthrough  PCopyVariant=Disabled  TRVariant=Disabled  FdbkBlocksVariant=Forward  IdealPFdbkVariant=Disabled  SatFdbkVariant=Disabled  DerivativeFilterVariant=ForwardEulerFilter  NVariant=InternalParameters  NCopyVariant=Disabled  FilterICVariant=InternalICsFilter  IntegratorICVariant=InternalICs  ExternalResetVariant=Disabled  TRSumVariant=Passthrough  SumFdbkVariant=Disabled  SumVariant=Sum_PID  TsampFilterVariant=InternalTs  TsampNgainVariant=Passthrough  TsampIntegralVariant=Disabled_SignalSpec  ExternalSaturationOutDataTypeStr=Inherit: Same as second input
      settings: LibrarySourceBlock=simulink/Discrete/Discrete PID Controller (2DOF)
  cfblk4 : simulink/Math Operations/MinMax Running Resettable  Function=min  vinit=0.0
  cfblk5 : Sum
  cfblk6 : Sqrt  Operator=rSqrt  AlgorithmType=Newton-Raphson
  cfblk7 : Subsystem
  cfblk9 : Delay  SampleTime=1
  cfblk2 : Outport
  wires:
  cfblk4/1 -> cfblk7/1(cfblk1), cfblk5/2
  cfblk5/1 -> cfblk2/1, cfblk10/1
  cfblk1/1 -> cfblk4/1
  cfblk6/1 -> cfblk3/2, cfblk9/1
  cfblk7/1(cfblk2) -> cfblk6/1
  cfblk8/1 -> cfblk3/1
  cfblk3/1 -> cfblk5/1
  cfblk9/1 -> cfblk7/3(cfblk13)
  cfblk10/1 -> cfblk7/2(cfblk12)
  cfblk7/2(cfblk14) -> cfblk11/1
  cfblk11/1 -> cfblk4/2

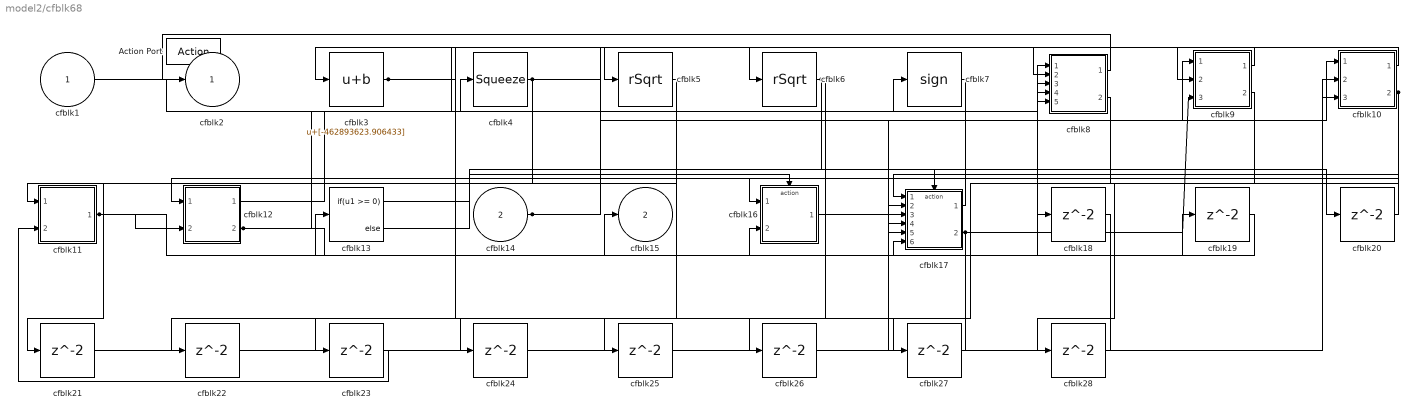
== system model2/cfblk68 ==
  cfblk1 : Inport
  cfblk14 : Inport  Port=2
  Action Port : ActionPort  ActionPortLabel=if(u1 >= 0)
  cfblk10 : Subsystem
  cfblk11 : Subsystem
  cfblk12 : Subsystem
  cfblk13 : If  IfExpression=u1 >= 0  SampleTime=1
  cfblk16 : Subsystem  TreatAsAtomicUnit=on
  cfblk17 : Subsystem  TreatAsAtomicUnit=on
  cfblk{18..28} (11 alike) : Delay
  cfblk3 : Bias  Bias=[-462893623.906433]  SaturateOnIntegerOverflow=off
  cfblk4 : Squeeze
  cfblk5 : Sqrt  Operator=rSqrt  AlgorithmType=Newton-Raphson
  cfblk6 : Sqrt  Operator=rSqrt  AlgorithmType=Newton-Raphson
  cfblk7 : Signum
  cfblk8 : Subsystem
  cfblk9 : Subsystem
  cfblk2 : Outport
  cfblk15 : Outport  Port=2
  wires:
  cfblk17/1(cfblk2) -> cfblk4/1
  cfblk7/1 -> cfblk16/1(cfblk1)
  cfblk4/1 -> cfblk9/2(cfblk8), cfblk20/1, cfblk21/1
  cfblk12/1(cfblk2) -> cfblk6/1
  cfblk12/2(cfblk10) -> cfblk8/1(cfblk1), cfblk8/4(cfblk14)
  cfblk3/1 -> cfblk5/1, cfblk27/1
  cfblk17/2(cfblk17) -> cfblk15/1, cfblk9/3(cfblk9), cfblk24/1
  cfblk11/1(cfblk2) -> cfblk12/2(cfblk9), cfblk18/1, cfblk19/1
  cfblk5/1 -> cfblk11/1(cfblk1)
  cfblk8/1(cfblk2) -> cfblk2/1
  cfblk10/1(cfblk2) -> cfblk3/1
  cfblk10/2(cfblk11) -> cfblk12/1(cfblk1), cfblk28/1
  cfblk16/1(cfblk2) -> cfblk10/1(cfblk1)
  cfblk9/1(cfblk2) -> cfblk8/2(cfblk12)
  cfblk6/1 -> cfblk25/1, cfblk26/1
  cfblk1/1 -> cfblk7/1
  cfblk14/1 -> cfblk8/3(cfblk13), cfblk9/1(cfblk1), cfblk8/5(cfblk15)
  cfblk13/1 -> cfblk16/Action
  cfblk13/2 -> cfblk17/Action
  cfblk18/1 -> cfblk16/2(cfblk9)
  cfblk19/1 -> cfblk17/6(cfblk16)
  cfblk20/1 -> cfblk17/1(cfblk1)
  cfblk21/1 -> cfblk17/3(cfblk13)
  cfblk8/2(cfblk16) -> cfblk22/1
  cfblk22/1 -> cfblk17/2(cfblk12)
  cfblk9/2(cfblk10) -> cfblk23/1
  cfblk23/1 -> cfblk11/2(cfblk16)
  cfblk24/1 -> cfblk10/3(cfblk10)
  cfblk25/1 -> cfblk10/2(cfblk9)
  cfblk26/1 -> cfblk17/5(cfblk15)
  cfblk27/1 -> cfblk17/4(cfblk14)
  cfblk28/1 -> cfblk13/1

== system model2/cfblk69 ==
  cfblk1 : Inport
  cfblk11 : Inport  Port=2
  cfblk12 : Inport  Port=3
  cfblk13 : Inport  Port=4
  Action Port : ActionPort  ActionPortLabel=else
  cfblk10 : Subsystem
  cfblk14 : Delay
  cfblk3 : DiscreteIntegrator  SampleTime=-1  ICPrevOutput=DiscIntNeverNeededParam  ICPrevScaledInput=DiscIntNeverNeededParam
  cfblk4 : Product
  cfblk5 : Sqrt  Operator=rSqrt  AlgorithmType=Newton-Raphson
  cfblk6 : Signum
  cfblk7 : Constant  Value=[-901741778.641720]  SampleTime=1
  cfblk8 : Constant  Value=[823575877.605597]  SampleTime=1
  cfblk9 : Subsystem
  cfblk2 : Outport
  wires:
  cfblk8/1 -> cfblk9/1(cfblk1)
  cfblk7/1 -> cfblk4/1
  cfblk13/1 -> cfblk3/1
  cfblk12/1 -> cfblk10/1(cfblk1)
  cfblk9/1(cfblk2) -> cfblk6/1
  cfblk3/1 -> cfblk4/2
  cfblk1/1 -> cfblk2/1
  cfblk10/1(cfblk2) -> cfblk5/1
  cfblk4/1 -> cfblk10/3(cfblk11)
  cfblk5/1 -> cfblk14/1
  cfblk14/1 -> cfblk10/2(cfblk10)

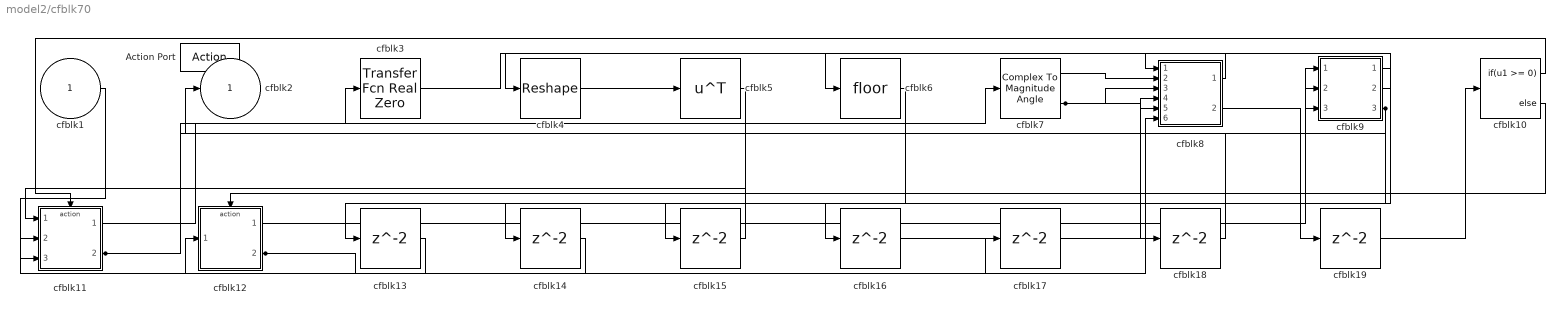
== system model2/cfblk70 ==
  cfblk1 : Inport
  Action Port : ActionPort  ActionPortLabel=if(u1 >= 0)
  cfblk10 : If  IfExpression=u1 >= 0  SampleTime=1
  cfblk11 : Subsystem  TreatAsAtomicUnit=on
  cfblk12 : Subsystem  TreatAsAtomicUnit=on
  cfblk{13..19} (7 alike) : Delay
  cfblk3 : simulink/Discrete/Transfer Fcn Real Zero  ZeroZ=0.75  ICPrevInput=0.0  DoSatur=off
  cfblk4 : Reshape
  cfblk5 : Math  Operator=transpose
  cfblk6 : Rounding
  cfblk7 : ComplexToMagnitudeAngle
  cfblk8 : Subsystem
  cfblk9 : Subsystem
  cfblk2 : Outport
  wires:
  cfblk8/1(cfblk2) -> cfblk4/1
  cfblk4/1 -> cfblk5/1
  cfblk12/1(cfblk2) -> cfblk9/1(cfblk1)
  cfblk9/2(cfblk16) -> cfblk6/1
  cfblk1/1 -> cfblk11/3(cfblk14)
  cfblk3/1 -> cfblk8/1(cfblk1)
  cfblk9/3(cfblk17) -> cfblk2/1, cfblk16/1
  cfblk7/1 -> cfblk8/2(cfblk11)
  cfblk7/2 -> cfblk8/3(cfblk12), cfblk9/3(cfblk15)
  cfblk11/1(cfblk2) -> cfblk3/1
  cfblk11/2(cfblk15) -> cfblk9/2(cfblk14), cfblk7/1
  cfblk12/2(cfblk13) -> cfblk17/1, cfblk18/1
  cfblk10/1 -> cfblk11/Action
  cfblk10/2 -> cfblk12/Action
  cfblk5/1 -> cfblk13/1
  cfblk13/1 -> cfblk12/1(cfblk1)
  cfblk9/1(cfblk2) -> cfblk14/1
  cfblk14/1 -> cfblk11/2(cfblk13)
  cfblk6/1 -> cfblk15/1
  cfblk15/1 -> cfblk11/1(cfblk1)
  cfblk16/1 -> cfblk8/6(cfblk15)
  cfblk17/1 -> cfblk8/4(cfblk13)
  cfblk18/1 -> cfblk8/5(cfblk14)
  cfblk8/2(cfblk16) -> cfblk19/1
  cfblk19/1 -> cfblk10/1

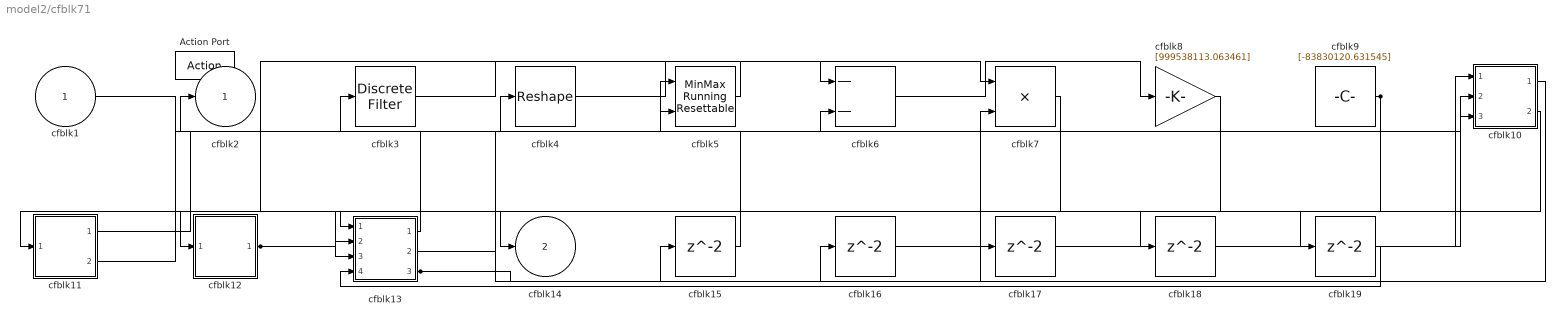
== system model2/cfblk71 ==
  cfblk1 : Inport
  Action Port : ActionPort  ActionPortLabel=else
  cfblk10 : Subsystem
  cfblk11 : Subsystem
  cfblk12 : Subsystem
  cfblk13 : Subsystem
  cfblk{15..19} (5 alike) : Delay
  cfblk3 : DiscreteFilter
  cfblk4 : Reshape
  cfblk5 : simulink/Math Operations/MinMax Running Resettable  Function=min  vinit=0.0
  cfblk6 : Sum  Inputs=--
  cfblk7 : Product
  cfblk8 : Gain  Gain=[999538113.063461]
  cfblk9 : Constant  Value=[-83830120.631545]  SampleTime=1
  cfblk2 : Outport
  cfblk14 : Outport  Port=2
  wires:
  cfblk12/1(cfblk2) -> cfblk18/1, cfblk19/1
  cfblk5/1 -> cfblk12/1(cfblk1)
  cfblk13/1(cfblk2) -> cfblk2/1
  cfblk9/1 -> cfblk13/1(cfblk1), cfblk13/3(cfblk10), cfblk5/2
  cfblk6/1 -> cfblk8/1
  cfblk1/1 -> cfblk3/1
  cfblk3/1 -> cfblk6/1
  cfblk7/1 -> cfblk11/1(cfblk1)
  cfblk11/1(cfblk2) -> cfblk6/2
  cfblk4/1 -> cfblk7/1
  cfblk8/1 -> cfblk14/1
  cfblk11/2(cfblk9) -> cfblk10/2(cfblk6)
  cfblk13/3(cfblk13) -> cfblk5/1, cfblk17/1
  cfblk10/2(cfblk8) -> cfblk13/2(cfblk9)
  cfblk10/1(cfblk2) -> cfblk15/1
  cfblk15/1 -> cfblk4/1
  cfblk13/2(cfblk12) -> cfblk16/1
  cfblk16/1 -> cfblk7/2
  cfblk17/1 -> cfblk10/3(cfblk7)
  cfblk18/1 -> cfblk10/1(cfblk1)
  cfblk19/1 -> cfblk13/4(cfblk11)

== system model2/cfblk72 ==
  cfblk1 : Inport
  Action Port : ActionPort  ActionPortLabel=if(u1 >= 0)
  cfblk3 : DiscreteFir
  cfblk4 : Bias  Bias=[987406145.129527]  SaturateOnIntegerOverflow=off
  cfblk5 : PermuteDimensions
  cfblk6 : Signum
  cfblk7 : Subsystem
  cfblk8 : Delay
  cfblk9 : Delay
  cfblk2 : Outport
  wires:
  cfblk1/1 -> cfblk3/1, cfblk7/4(cfblk14)
  cfblk4/1 -> cfblk5/1
  cfblk3/1 -> cfblk7/1(cfblk1), cfblk2/1
  cfblk5/1 -> cfblk8/1, cfblk9/1
  cfblk7/1(cfblk2) -> cfblk6/1
  cfblk6/1 -> cfblk4/1
  cfblk8/1 -> cfblk7/2(cfblk12)
  cfblk9/1 -> cfblk7/3(cfblk13)

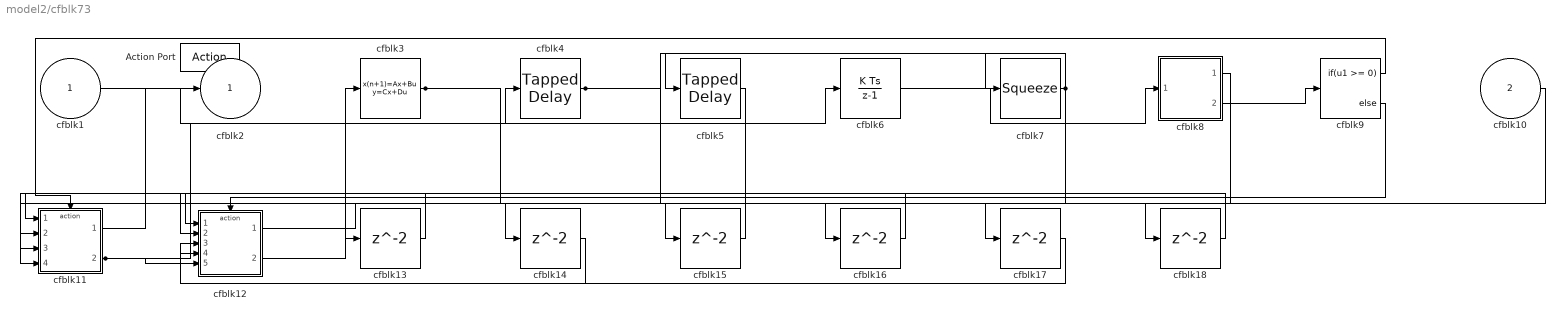
== system model2/cfblk73 ==
  cfblk1 : Inport
  cfblk10 : Inport  Port=2
  Action Port : ActionPort  ActionPortLabel=else
  cfblk11 : Subsystem  TreatAsAtomicUnit=on
  cfblk12 : Subsystem  TreatAsAtomicUnit=on
  cfblk{13..18} (6 alike) : Delay
  cfblk3 : DiscreteStateSpace  SampleTime=-1
  cfblk4 : simulink/Discrete/Tapped Delay  vinit=0.0  samptime=-1  NumDelays=1  DelayOrder=Oldest  includeCurrent=off
  cfblk5 : simulink/Discrete/Tapped Delay  vinit=0.0  samptime=-1  NumDelays=1  DelayOrder=Oldest  includeCurrent=off
  cfblk6 : DiscreteIntegrator  SampleTime=-1  ICPrevOutput=DiscIntNeverNeededParam  ICPrevScaledInput=DiscIntNeverNeededParam
  cfblk7 : Squeeze
  cfblk8 : Subsystem
  cfblk9 : If  IfExpression=u1 >= 0  SampleTime=1
  cfblk2 : Outport
  wires:
  cfblk11/1(cfblk2) -> cfblk2/1
  cfblk11/2(cfblk10) -> cfblk4/1, cfblk12/5(cfblk13)
  cfblk10/1 -> cfblk11/3(cfblk8)
  cfblk7/1 -> cfblk5/1, cfblk14/1
  cfblk8/1(cfblk2) -> cfblk11/4(cfblk9)
  cfblk6/1 -> cfblk8/1(cfblk1)
  cfblk1/1 -> cfblk6/1
  cfblk8/2(cfblk15) -> cfblk9/1
  cfblk12/2(cfblk14) -> cfblk3/1
  cfblk4/1 -> cfblk7/1, cfblk18/1
  cfblk3/1 -> cfblk16/1, cfblk17/1
  cfblk9/1 -> cfblk11/Action
  cfblk9/2 -> cfblk12/Action
  cfblk5/1 -> cfblk13/1
  cfblk13/1 -> cfblk11/2(cfblk7)
  cfblk14/1 -> cfblk12/4(cfblk12)
  cfblk12/1(cfblk2) -> cfblk15/1
  cfblk15/1 -> cfblk11/1(cfblk1)
  cfblk16/1 -> cfblk12/1(cfblk1)
  cfblk17/1 -> cfblk12/3(cfblk11)
  cfblk18/1 -> cfblk12/2(cfblk10)

== system model2/cfblk74 ==
  cfblk1 : Inport
  cfblk10 : Inport  Port=2
  cfblk11 : Inport  Port=3
  Action Port : ActionPort  ActionPortLabel=if(u1 >= 0)
  cfblk13 : Delay
  cfblk3 : slpidlib/PID Controller  Controller=PID  Form=Parallel  TimeDomain=Discrete-time  UseExternalTs=off  SampleTime=-1  IntegratorMethod=Forward Euler  FilterMethod=Forward Euler  ControllerParametersSource=internal  P=1  I=1  UseKiTs=off  D=0  N=100  UseFilter=on  TunerSelectOption=Transfer Function Based (PID Tuner App)  InitialConditionSource=internal  InitialConditionForIntegrator=0  InitialConditionForFilter=0  DifferentiatorICPrevScaledInput=0  ExternalReset=none  TrackingMode=off  Kt=1  LimitOutput=off  SatLimitsSource=internal  UpperSaturationLimit=inf  LowerSaturationLimit=-inf  LinearizeAsGain=off  AntiWindupMode=none  Kb=1  LimitIntegrator=off  UpperIntegratorSaturationLimit=inf  LowerIntegratorSaturationLimit=-inf  POutMin=[]  POutMax=[]  IOutMin=[]  IOutMax=[]  DOutMin=[]  DOutMax=[]  NOutMin=[]  NOutMax=[]  SumOutMin=[]  SumOutMax=[]  SaturationOutMin=[]  SaturationOutMax=[]  PParamMin=[]  PParamMax=[]  IParamMin=[]  IParamMax=[]  DParamMin=[]  DParamMax=[]  NParamMin=[]  NParamMax=[]  KbParamMin=[]  KbParamMax=[]  KtParamMin=[]  KtParamMax=[]  KbOutMin=[]  KbOutMax=[]  KtOutMin=[]  KtOutMax=[]  IntegratorOutMin=[]  IntegratorOutMax=[]  FilterOutMin=[]  FilterOutMax=[]  SumI1OutMin=[]  SumI1OutMax=[]  SumI2OutMin=[]  SumI2OutMax=[]  SumI3OutMin=[]  SumI3OutMax=[]  SumI4OutMin=[]  SumI4OutMax=[]  SumDOutMin=[]  SumDOutMax=[]  DifferentiatorOutMin=[]  DifferentiatorOutMax=[]  FilterDiffOutCoefMin=[]  FilterDiffOutCoefMax=[]  ReciprocalOutMin=[]  ReciprocalOutMax=[]  SumDenOutMin=[]  SumDenOutMax=[]  SumNumOutMin=[]  SumNumOutMax=[]  DivideOutMin=[]  DivideOutMax=[]  UdiffTsProdOutMin=[]  UdiffTsProdOutMax=[]  NTsProdOutMin=[]  NTsProdOutMax=[]  UintegralTsProdOutMin=[]  UintegralTsProdOutMax=[]  UngainTsProdOutMin=[]  UngainTsProdOutMax=[]  ClampingZeroOutDataTypeStr=Inherit: Inherit via back propagation  ClampingZeroOutMin=[]  ClampingZeroOutMax=[]  FilterDenConstantOutDataTypeStr=Inherit: Inherit via back propagation  FilterDenConstantOutMin=[]  FilterDenConstantOutMax=[]  PCopyOutDataTypeStr=Inherit: Inherit via back propagation  PCopyOutMin=[]  PCopyOutMax=[]  NCopyOutDataTypeStr=Inherit: Inherit via back propagation  NCopyOutMin=[]  NCopyOutMax=[]  IntegratorContinuousStateAttributes=''  IntegratorStateMustResolveToSignalObject=off  IntegratorRTWStateStorageClass=Auto  FilterContinuousStateAttributes=''  FilterStateMustResolveToSignalObject=off  FilterRTWStateStorageClass=Auto  ParallelPVariant=InternalParameters  IdealPVariant=Disabled  IVariant=InternalParameters  DVariant=InternalParameters  IntegratorVariant=Discrete  SatVariant=Disabled  AWVariant=Passthrough  PCopyVariant=Disabled  TRVariant=Disabled  FdbkBlocksVariant=Forward  IdealPFdbkVariant=Disabled  SatFdbkVariant=Disabled  DerivativeFilterVariant=ForwardEulerFilter  NVariant=InternalParameters  NCopyVariant=Disabled  FilterICVariant=InternalICsFilter  IntegratorICVariant=InternalICs  ExternalResetVariant=Disabled  TRSumVariant=Passthrough  SumFdbkVariant=Disabled  SumVariant=Sum_PID  TsampFilterVariant=InternalTs  TsampNgainVariant=Passthrough  TsampIntegralVariant=Disabled_SignalSpec  ExternalSaturationOutDataTypeStr=Inherit: Same as second input
      settings: LibrarySourceBlock=simulink/Discrete/Discrete PID Controller
  cfblk4 : DiscreteFir
  cfblk5 : MinMax  Function=max  Inputs=2
  cfblk6 : ComplexToMagnitudeAngle
  cfblk7 : ComplexToMagnitudeAngle
  cfblk8 : Abs  SaturateOnIntegerOverflow=off
  cfblk9 : Sum  Inputs=|++
  cfblk2 : Outport
  cfblk12 : Outport  Port=2
  wires:
  cfblk1/1 -> cfblk5/2
  cfblk4/1 -> cfblk7/1
  cfblk5/1 -> cfblk3/1
  cfblk11/1 -> cfblk6/1
  cfblk6/1 -> cfblk12/1
  cfblk10/1 -> cfblk8/1
  cfblk6/2 -> cfblk4/1
  cfblk7/1 -> cfblk9/1
  cfblk7/2 -> cfblk2/1
  cfblk8/1 -> cfblk9/2
  cfblk3/1 -> cfblk13/1
  cfblk13/1 -> cfblk5/1
